simulink model "lqg_demo"  (R2014a)
settings: Solver=ode45  StartTime=0.0  StopTime=10.0  RelTol=1e-3
values from neighbouring files (symbols this model uses):
  A = 2.2    [PBA1_script.m]    (also in PBA3_1.m = simplify(subs(jacobian(F_x, x), x_T, equ)); cruise_control.m; gyro_pendulum.m = simplify(subs(jacobian(F_x, x), x_T, equ)); helicopter_eom.m = [A11, A12; A21])
  A_m = A    [sim_params.m]
  B = simplify(subs(jacobian(F_x, F), x_T, equ))    [PBA3_1.m]    (also in gyro_pendulum.m = simplify(subs(jacobian(F_x, t), x_T, equ)); helicopter_eom.m = [B11; B21]; massandcart.m = simplify(eval(Jacu)); sim_params.m = [0; 1])
  B_m = B    [sim_params.m]
  C = 50    [Tute2Q3.m]    (also in helicopter_eom.m = [eye(3), zeros(3,3)]; predprey.m; sim_params.m = [1 0])
  C_m = C    [sim_params.m]
  Q = -eye(2)    [PBA2_2_2script.m]    (also in PBA2_2_3script.m; PBA2_2_script.m; extended_kalman_filter.m = 0.1*eye(6); helicopter_eom.m = [Q1, Q2, Q3])
  R = 0.5*eye(3)    [extended_kalman_filter.m]    (also in sim_params.m = 0.1)
settings Model: Creator=uqmkearn  LastModifiedBy=uqmkearn

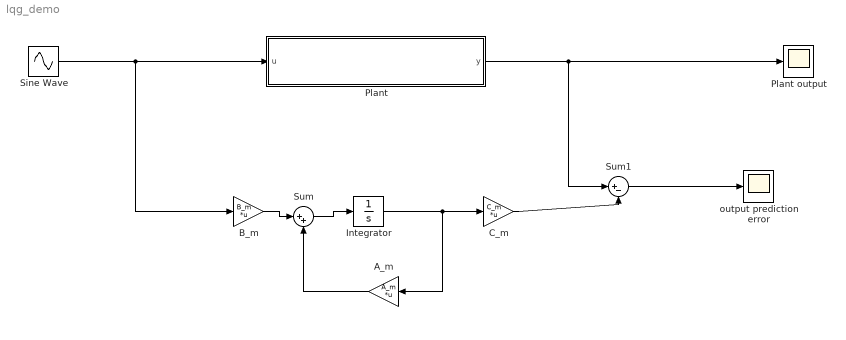
== system lqg_demo ==
  A_m : Gain  Gain=A_m  Multiplication=Matrix(K*u)
  B_m : Gain  Gain=B_m  Multiplication=Matrix(K*u)
  C_m : Gain  Gain=C_m  Multiplication=Matrix(K*u)
  Integrator : Integrator  InitialCondition=[0.5 0.5]'
  Plant : Subsystem
  Plant output : Scope
  Sine Wave : Sin  SampleTime=0
  Sum : Sum  Inputs=|++
  Sum1 : Sum  Inputs=|+-
  output prediction error : Scope
  wires:
  Plant/1(y) -> Sum1/1, Plant output/1
  Integrator/1 -> A_m/1, C_m/1
  B_m/1 -> Sum/1
  A_m/1 -> Sum/2
  Sum/1 -> Integrator/1
  C_m/1 -> Sum1/2
  Sum1/1 -> output prediction error/1
  Sine Wave/1 -> B_m/1, Plant/1(u)

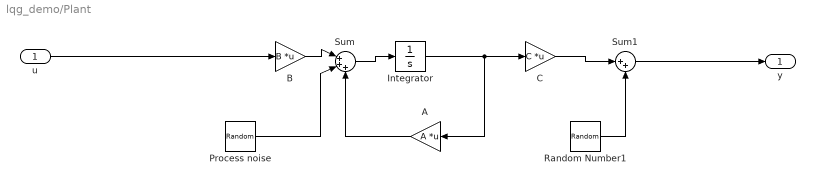
== system lqg_demo/Plant ==
  u : Inport
  A : Gain  Gain=A  Multiplication=Matrix(K*u)
  B : Gain  Gain=B  Multiplication=Matrix(K*u)
  C : Gain  Gain=C  Multiplication=Matrix(K*u)
  Integrator : Integrator  InitialCondition=[0.5 0.5]'
  Process noise : RandomNumber  Mean=zeros(size(A,2),1)  Variance=diag(Q)  SampleTime=0.1
  Random Number1 : RandomNumber  Mean=zeros(size(C,1),1)  Variance=diag(R)  SampleTime=0.1
  Sum : Sum  Inputs=|+++
  Sum1 : Sum  Inputs=|++
  y : Outport
  wires:
  Random Number1/1 -> Sum1/2
  Sum1/1 -> y/1
  Integrator/1 -> A/1, C/1
  B/1 -> Sum/1
  u/1 -> B/1
  Process noise/1 -> Sum/2
  C/1 -> Sum1/1
  A/1 -> Sum/3
  Sum/1 -> Integrator/1
